simulink model "VTC6_Sim"  (R2019b)
settings: Solver=FixedStepAuto  StartTime=time(1)  StopTime=time(end)  FixedStep=0.005  RelTol=1e-3
values from neighbouring files (symbols this model uses):
  C1_lut = [0 0 0 0 0 0 126.994699088 352.457442321 497.419117814 604.150647217 682.181489366 724.029150077 ... (4000 elements, 100x40)]    [Lut_Sim.mat]
  C2_lut = [0 0 0 0 0 0 0 0 2740.78189782 4641.58158357 6032.60446044 7596.33080038 ... (4000 elements, 100x40)]    [Lut_Sim.mat]
  OCV_lut = [2.54020422692 2.68040845384 2.81538392295 2.88895607028 2.94916911681 2.99822851777 3.0372449808 3.07029327569 3.09992793679 3.12541619029 3.15027805329 3.1746347997 ... (100 elements, 100x1)]    [Lut_Sim.mat]
  R0_lut = [0.0362413738386 0.0362203254133 0.0361868714515 0.0360332906417 0.03531504612 0.033997800577 0.0321878921394 0.0300582863978 0.0278565656259 0.0260239150176 0.0249802665838 0.0249284563175 ... (4000 elements, 100x40)]    [Lut_Sim.mat]
  R1_lut = [0.215925261746 0.171921338964 0.129792738987 0.0931470250311 0.0719266383986 0.0638366906305 0.062733914906 0.0618460989873 0.0564806765835 0.0499255430523 0.046971743749 0.0498114830758 ... (4000 elements, 100x40)]    [Lut_Sim.mat]
  R2_lut = [0.0719609328313 0.0632939846071 0.0550915881819 0.0480256894637 0.0435514337082 0.0413049054741 0.0403227924517 0.0395210290499 0.0381406969202 0.0367986580468 0.0362103816205 0.0362217699629 ... (4000 elements, 100x40)]    [Lut_Sim.mat]
  SOC_lut = [0 2.91262135922 3.21380154603 3.51498173285 3.831220929 4.26793219987 4.68205495674 4.98323514355 5.39735790041 5.84912818063 6.37619350755 6.97855388117 ... (117 elements, 117x1)]    [Lut_Sim.mat]
undefined symbols (not defined in the file or in its folder): Voltage
libraries: nesl_utility x12, fl_lib x10, ee_lib x2
settings Model: OrderedModelArguments=off  Creator=Utente  LastModifiedBy=PcElettronicaDynamis
settings DataIOCC: SaveOutput=off  DSMLogging=off  InspectSignalLogs=on  OutputOption=AdditionalOutputTimes  OutputTimes=SDO_OutputTimes  ReturnWorkspaceOutputsName=SimOut

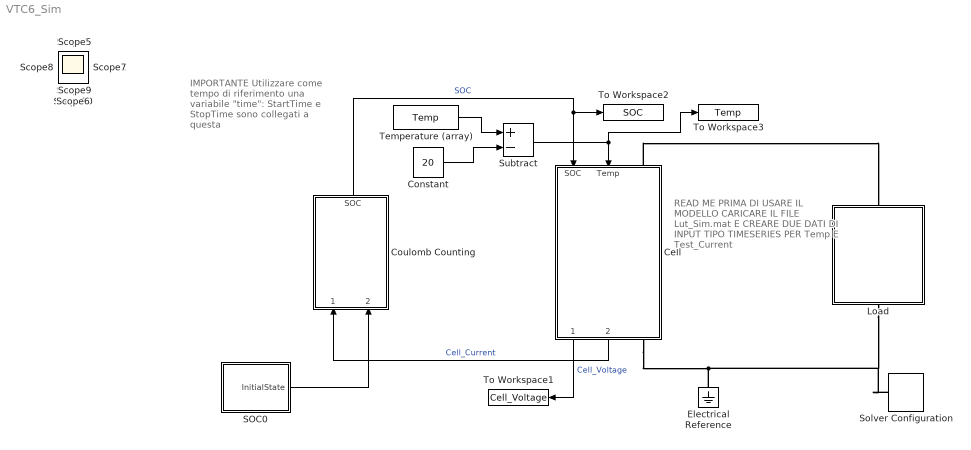
== system VTC6_Sim ==
  note: IMPORTANTE
      | Utilizzare come tempo di riferimento una variabile "time": StartTime e StopTime sono collegati a questa
  note: READ ME
      | PRIMA DI USARE IL MODELLO CARICARE IL FILE Lut_Sim.mat E CREARE DUE DATI DI INPUT TIPO TIMESERIES PER Temp E Test_Current
  Cell : Subsystem
  Constant : Constant  Value=20  SampleTime=0.005
  Coulomb Counting : Subsystem
  Electrical Reference : fl_lib/Electrical/Electrical Elements/Electrical Reference
  Load : Subsystem
  SOC0 : Subsystem
  Solver Configuration : nesl_utility/Solver Configuration  PhysicalDomain=network_engine_domain  SubClassName=solver  LeftPortType=input  RightPortType=generic  Tones=[]  Harmonics=[]  SimulateNoise=off  Profile=off  UseLocalSampling=off  EnableSwitchedLinearOptims=on  FrequencyDomain=off  UseCCode=off  RelTol=0.001  AbsTol=1e-06  MinStep=1e-09  ToWorkspace=off  RevertToSquareIcSolve=off  NumHomotopyIterations=100  PhasorMode=off  PhasorModeNumHarmonics=1  DoDC=off  ResidualTolerance=1e-09  UseLocalSolver=off  LocalSolverChoice=NE_BACKWARD_EULER_ADVANCER  LocalSolverSampleTime=0.001  DoFixedCost=off  MaxNonlinIter=3  MaxModeIter=2  LinearAlgebra=auto  EquationFormulation=NE_TIME_EF  DelaysMemoryBudget=1024  AutomaticFiltering=on  FilteringTimeConstant=0.001  PartitionStorageMethod=AS_NEEDED  PartitionMemoryBudget=1024  PartitionMethod=ROBUST
  Subtract : Sum  Inputs=+-
  Temperature (array) : FromWorkspace  VariableName=Temp  SampleTime=0.005
  To Workspace1 : ToWorkspace  VariableName=Cell_Voltage  SaveFormat=Timeseries  SampleTime=0.005
  To Workspace2 : ToWorkspace  VariableName=SOC  SaveFormat=Timeseries  SampleTime=0.005
  To Workspace3 : ToWorkspace  VariableName=Temp  SaveFormat=Timeseries  SampleTime=0.005
  Scope{,1..10} (11 alike) : Scope
  wires:
  Cell/2(Cell_Current) -> Coulomb Counting/1(Cell_Current)  "Cell_Current"
  Coulomb Counting/1(SOC) -> Cell/1(SOC), To Workspace2/1  "SOC"
  Cell/1(Cell_Voltage) -> To Workspace1/1  "Cell_Voltage"
  SOC0/1(InitialState) -> Coulomb Counting/2(InitialState)
  Temperature (array)/1 -> Subtract/1
  Constant/1 -> Subtract/2
  Subtract/1 -> To Workspace3/1, Cell/2(Temp)
  connections:
  Electrical Reference/LConn1 -- Cell/RConn1 -- Solver Configuration/RConn1 -- Load/LConn1
  Cell/LConn1 -- Load/RConn1

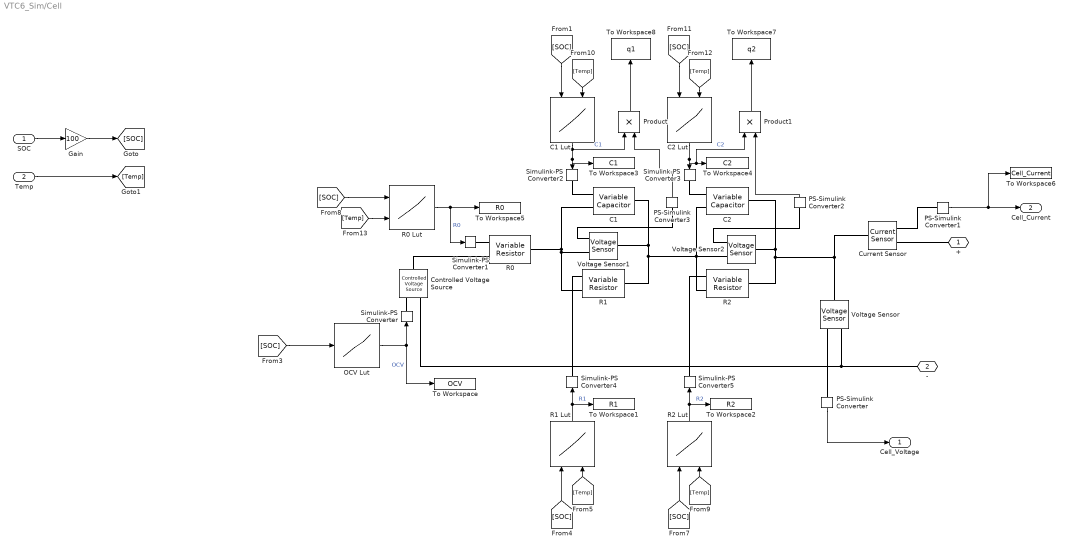
== system VTC6_Sim/Cell ==
  SOC : Inport  SampleTime=0.05
  Temp : Inport  Port=2  SampleTime=0.05
  C1 : ee_lib/Passive/Variable Capacitor  prm=2  Cmin=1e-9 F  r=1e-6 Ohm  v0=0 V  q0=0 C
      settings: SourceProductName=Simscape Electrical  SourceProductBaseCode=PS  InternalSimscapePortConfiguration="{\"Bottom\":[],\"Left\":[{\"id\":\"C\",\"label\":\"C\",\"type\":\"input\"},{\"id\":\"p\",\"label\":\"+\",\"type\":\"foundation.electrical.electrical\"}],\"Right\":[{\"id\":\"n\",\"label\":\"-\",\"type\":\"foundation.electrical.electrical\"}],\"Top\":[]}"
  C1 Lut : Lookup_n-D  BreakpointsForDimension1=[1:100]  BreakpointsForDimension2=[1:40]  Table=C1_lut  RndMeth=Simplest  InputSameDT=on
  C2 : ee_lib/Passive/Variable Capacitor  prm=2  Cmin=1e-9 F  r=1e-6 Ohm  v0=0 V  q0=0 C
      settings: SourceProductName=Simscape Electrical  SourceProductBaseCode=PS  InternalSimscapePortConfiguration="{\"Bottom\":[],\"Left\":[{\"id\":\"C\",\"label\":\"C\",\"type\":\"input\"},{\"id\":\"p\",\"label\":\"+\",\"type\":\"foundation.electrical.electrical\"}],\"Right\":[{\"id\":\"n\",\"label\":\"-\",\"type\":\"foundation.electrical.electrical\"}],\"Top\":[]}"
  C2 Lut : Lookup_n-D  BreakpointsForDimension1=[1:100]  BreakpointsForDimension2=[1:40]  Table=C2_lut  RndMeth=Simplest  InputSameDT=on
  Controlled Voltage Source : fl_lib/Electrical/Electrical Sources/Controlled Voltage Source
  Current Sensor : fl_lib/Electrical/Electrical Sensors/Current Sensor
  Gain : Gain  Gain=100
  OCV Lut : Lookup_n-D  NumberOfTableDimensions=1  BreakpointsForDimension1=[1:100]  Table=OCV_lut  InternalRulePriority=Speed  RndMeth=Simplest  InputSameDT=on
  PS-Simulink Converter{,1..3} (4 alike) : nesl_utility/PS-Simulink Converter  PhysicalDomain=network_engine_domain  SubClassName=ps_output  LeftPortType=input  RightPortType=output  PseudoPeriodic=off  Frequencies=[]  Unit=inherit  AffineConversion=off
  Product : Product
  Product1 : Product
  R0 : fl_lib/Electrical/Electrical Elements/Variable Resistor  Rmin=0 Ohm  i_specify=off  i_priority=None  i=0 A  i_nominal_specify=off  i_nominal_unit=A  i_nominal_value=1  v_specify=off  v_priority=None  v=0 V  v_nominal_specify=off  v_nominal_unit=V  v_nominal_value=1
  "R0 Lut " : Lookup_n-D  BreakpointsForDimension1=[1:100]  BreakpointsForDimension2=[1:40]  Table=R0_lut  RndMeth=Simplest  InputSameDT=on
  R1 : fl_lib/Electrical/Electrical Elements/Variable Resistor  Rmin=0 Ohm  i_specify=off  i_priority=None  i=0 A  i_nominal_specify=off  i_nominal_unit=A  i_nominal_value=1  v_specify=off  v_priority=None  v=0 V  v_nominal_specify=off  v_nominal_unit=V  v_nominal_value=1
  R1 Lut : Lookup_n-D  BreakpointsForDimension1=[1:100]  BreakpointsForDimension2=[1:40]  Table=R1_lut  RndMeth=Simplest  InputSameDT=on
  R2 : fl_lib/Electrical/Electrical Elements/Variable Resistor  Rmin=0 Ohm  i_specify=off  i_priority=None  i=0 A  i_nominal_specify=off  i_nominal_unit=A  i_nominal_value=1  v_specify=off  v_priority=None  v=0 V  v_nominal_specify=off  v_nominal_unit=V  v_nominal_value=1
  R2 Lut : Lookup_n-D  BreakpointsForDimension1=[1:100]  BreakpointsForDimension2=[1:40]  Table=R2_lut  RndMeth=Simplest  InputSameDT=on
  Simulink-PS Converter{,1..5} (6 alike) : nesl_utility/Simulink-PS Converter  PhysicalDomain=network_engine_domain  SubClassName=ps_input  LeftPortType=input  RightPortType=output  PseudoPeriodic=off  Frequencies=[]  NoiseDistribution=none  NoiseParameters=[]  Unit=1  AffineConversion=off  FilteringAndDerivatives=provide  SimscapeFilterOrder=1  InputFilterTimeConstant=0.001  UdotUserProvided=0
  To Workspace : ToWorkspace  VariableName=OCV  SaveFormat=Timeseries  SampleTime=0.005
  To Workspace1 : ToWorkspace  VariableName=R1  SaveFormat=Timeseries  SampleTime=0.005
  To Workspace2 : ToWorkspace  VariableName=R2  SaveFormat=Timeseries  SampleTime=0.005
      settings: MaxDataPoints=Inf
  To Workspace3 : ToWorkspace  VariableName=C1  SaveFormat=Timeseries  SampleTime=0.005
  To Workspace4 : ToWorkspace  VariableName=C2  SaveFormat=Timeseries  SampleTime=0.005
  To Workspace5 : ToWorkspace  VariableName=R0  SaveFormat=Timeseries  SampleTime=0.005
  To Workspace6 : ToWorkspace  VariableName=Cell_Current  SaveFormat=Timeseries  SampleTime=0.005
  To Workspace7 : ToWorkspace  VariableName=q2  SaveFormat=Timeseries  SampleTime=-1
  To Workspace8 : ToWorkspace  VariableName=q1  SaveFormat=Timeseries  SampleTime=-1
  Voltage Sensor : fl_lib/Electrical/Electrical Sensors/Voltage Sensor
  Voltage Sensor1 : fl_lib/Electrical/Electrical Sensors/Voltage Sensor
  Voltage Sensor2 : fl_lib/Electrical/Electrical Sensors/Voltage Sensor
  + : PMIOPort  Side=Left
  - : PMIOPort  Port=2  Side=Right
  Cell_Voltage : Outport  SampleTime=0.05
  Cell_Current : Outport  Port=2  SampleTime=0.05
  wires:
  PS-Simulink Converter/1 -> Cell_Voltage/1
  R1 Lut/1 -> To Workspace1/1, Simulink-PS Converter4/1  "R1"
  OCV Lut/1 -> To Workspace/1, Simulink-PS Converter/1  "OCV"
  "R0 Lut "/1 -> To Workspace5/1, Simulink-PS Converter1/1  "R0"
  R2 Lut/1 -> Simulink-PS Converter5/1, To Workspace2/1  "R2"
  Temp/1 -> [Temp]
  PS-Simulink Converter1/1 -> To Workspace6/1, Cell_Current/1
  Gain/1 -> [SOC]
  C2 Lut/1 -> Product1/1, To Workspace4/1, Simulink-PS Converter3/1  "C2"
  C1 Lut/1 -> Simulink-PS Converter2/1, To Workspace3/1, Product/1  "C1"
  [SOC] -> OCV Lut/1
  SOC/1 -> Gain/1
  [Temp] -> C1 Lut/2
  [SOC] -> C1 Lut/1
  [Temp] -> C2 Lut/2
  [SOC] -> C2 Lut/1
  [Temp] -> R1 Lut/2
  [SOC] -> R1 Lut/1
  [Temp] -> R2 Lut/2
  [SOC] -> R2 Lut/1
  PS-Simulink Converter3/1 -> Product/2
  PS-Simulink Converter2/1 -> Product1/2
  [Temp] -> "R0 Lut "/2
  [SOC] -> "R0 Lut "/1
  Product1/1 -> To Workspace7/1
  Product/1 -> To Workspace8/1
  connections:
  C2/LConn2 -- C1/RConn1 -- Voltage Sensor1/LConn1 -- R1/RConn1 -- Voltage Sensor2/RConn2 -- R2/LConn2
  Voltage Sensor/LConn1 -- Voltage Sensor2/LConn1 -- C2/RConn1 -- R2/RConn1 -- Current Sensor/LConn1
  R0/RConn1 -- Voltage Sensor1/RConn2 -- R1/LConn2 -- C1/LConn2
  Simulink-PS Converter3/RConn1 -- C2/LConn1
  Controlled Voltage Source/RConn2 -- Voltage Sensor/RConn2 -- -/RConn1
  Simulink-PS Converter5/RConn1 -- R2/LConn1
  PS-Simulink Converter/LConn1 -- Voltage Sensor/RConn1
  Simulink-PS Converter2/RConn1 -- C1/LConn1
  Simulink-PS Converter1/RConn1 -- R0/LConn1
  R1/LConn1 -- Simulink-PS Converter4/RConn1
  Simulink-PS Converter/RConn1 -- Controlled Voltage Source/RConn1
  Controlled Voltage Source/LConn1 -- R0/LConn2
  PS-Simulink Converter1/LConn1 -- Current Sensor/RConn1
  Current Sensor/RConn2 -- +/RConn1
  PS-Simulink Converter2/LConn1 -- Voltage Sensor2/RConn1
  PS-Simulink Converter3/LConn1 -- Voltage Sensor1/RConn1

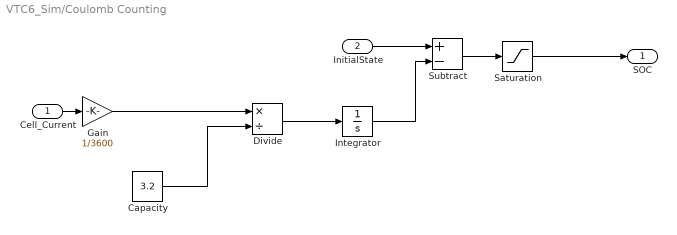
== system VTC6_Sim/Coulomb Counting ==
  Cell_Current : Inport  SampleTime=0.05
  InitialState : Inport  Port=2
  Capacity : Constant  Value=3.2
  Divide : Product  Inputs=*/
  Gain : Gain  Gain=1/3600
  Integrator : Integrator
  Saturation : Saturate  UpperLimit=1  LowerLimit=0
  Subtract : Sum  Inputs=+-
  SOC : Outport  SampleTime=0.05  VectorParamsAs1DForOutWhenUnconnected=off
  wires:
  Divide/1 -> Integrator/1
  Cell_Current/1 -> Gain/1
  Subtract/1 -> Saturation/1
  Integrator/1 -> Subtract/2
  Capacity/1 -> Divide/2
  InitialState/1 -> Subtract/1
  Saturation/1 -> SOC/1
  Gain/1 -> Divide/1

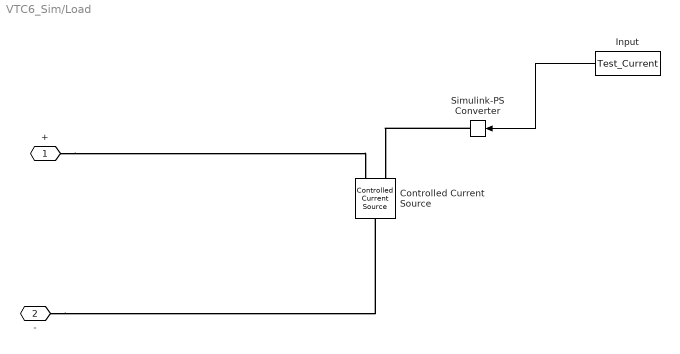
== system VTC6_Sim/Load ==
  Controlled Current Source : fl_lib/Electrical/Electrical Sources/Controlled Current Source
  Input : FromWorkspace  VariableName=Test_Current  SampleTime=0.005
  Simulink-PS Converter : nesl_utility/Simulink-PS Converter  PhysicalDomain=network_engine_domain  SubClassName=ps_input  LeftPortType=input  RightPortType=output  PseudoPeriodic=off  Frequencies=[]  NoiseDistribution=none  NoiseParameters=[]  Unit=1  AffineConversion=off  FilteringAndDerivatives=provide  SimscapeFilterOrder=1  InputFilterTimeConstant=0.001  UdotUserProvided=0
  + : PMIOPort  Side=Right
  - : PMIOPort  Port=2  Side=Left
  wires:
  Input/1 -> Simulink-PS Converter/1
  connections:
  +/RConn1 -- Controlled Current Source/RConn2
  Simulink-PS Converter/RConn1 -- Controlled Current Source/RConn1
  -/RConn1 -- Controlled Current Source/LConn1

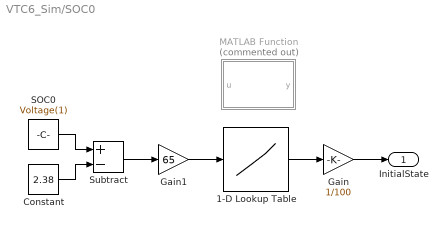
== system VTC6_Sim/SOC0 ==
  1-D Lookup Table : Lookup_n-D  NumberOfTableDimensions=1  BreakpointsForDimension1=[1:117]  Table=SOC_lut  InternalRulePriority=Speed  RndMeth=Simplest  InputSameDT=on
  Constant : Constant  Value=2.38  SampleTime=0.005
  Gain : Gain  Gain=1/100
  Gain1 : Gain  Gain=65
  MATLAB Function : MATLAB Function  Commented=on  TreatAsAtomicUnit=on
  SOC0 : Constant  Value=Voltage(1)  SampleTime=0.005
  Subtract : Sum  Inputs=+-
  InitialState : Outport
  wires:
  1-D Lookup Table/1 -> Gain/1
  Gain/1 -> InitialState/1
  Gain1/1 -> 1-D Lookup Table/1
  Subtract/1 -> Gain1/1
  SOC0/1 -> Subtract/1
  Constant/1 -> Subtract/2

== matlab function VTC6_Sim/SOC0/MATLAB Function ==
  data: u input; y output
function y = setState(u)
y = 0;
y(1,1) = interp1(sococv(1:117,2), sococv(1:117,1), u);

end
